simulink model "hilTest"  (R2019b)
settings: Solver=ode1  StartTime=0.0  StopTime=Inf  FixedStep=0.001  RelTol=1e-3
PostLoadFcn:
  | , if any(exist('dsrtsu_mdlpostloadfcn', 'file') ~= 0), dsrtsu_mdlpostloadfcn('Execute', bdroot); end,
InitFcn:
  | , if any(exist('rtifpga_mdlclblib', 'file') ~= 0), rtifpga_mdlclblib('Init', bdroot); end,
undefined symbols (not defined in the file or in its folder): rticanmm_blockfcn, rticanmm_initfcn
libraries: rtimmsu_dsrtlib x2
Description:
  | Standard RTI1006 template.
  | Supported MATLAB version:  R2019b.
settings Model: Tag=RTI1006  DSRTSU_INTERNAL_RTI_VER=560  DSRTSU_INTERNAL_RTI_TYPE=rti1006  RTICANMMDATA=struct('GeneralSetupData',struct('modelroot','C:\Users\uweco\Desktop\Git\ArudinoCANDisplay\HIL','generalsettings',struct('filesettings',struct('destfolder',struct('Name','RTICANMM_FILES','Check',1),'buildfolder',struct('Name','.','Check',1),'AbsDestfolder',struct('Name','C:\Users\uweco\Desktop\Git\ArudinoCANDisplay\HIL\RTICANMM_FILES'),'AbsBuildfolder',struct('Name','C:\Users\uweco\Desktop\Git\ArudinoCANDisplay\HIL'))),'options',struct('addpaths',1,'rmpaths',1,'addtrcexclusion',1,'cannavigator',struct('checkmonitoring',1),'show_usrtrc',0,'use_usrtrc',0,'addpath2usrmk',1,'disableclosing',0),'advanced',struct('options',ones(1,100)),'MPSetup',{{}},'modelname','hilTest','blockdata',struct('generalsettings',struct('filesettings',struct('destfolder',struct('Name','.','Check',1),'AbsDestfolder',struct('Name','T:\TOOL_SOURCES\CANnedy\m'),'buildfolder',struct('Name','.','Check',1),'AbsBuildfolder',struct('Name','C:\MATLAB6p5\work'))),'options',struct('addpaths',1,'rmpaths',1,'addpath2usrmk',1),'modelname','rticanmmlib','modelroot','T:\TOOL_SOURCES\CANnedy\m'),'MMType','RTICANMM','block',['hilTest/RTICANMM' char(10) 'GeneralSetup'],'RTI',struct('Type','RTI1006','Ver','7.14','Date','02-May-2020'),'version','5.4.737888.359837963','userdata',struct('HostServiceChannelID',{{'CAVPCM'}})))  DSRTSU_INTERNAL_RTIFPGA=160  Creator=uweco  LastModifiedBy=uweco
settings DataIOCC: ReturnWorkspaceOutputs=off
settings OptimizationCC: BlockReduction=off  OptimizeBlockIOStorage=off  BufferReuse=off  GlobalBufferReuse=off  ExpressionFolding=off  LocalBlockOutputs=off  OptimizeDataStoreBuffers=off  BusAssignmentInplaceUpdate=off
settings DebuggingCC: PregeneratedLibrarySubsystemCodeDiagnostic=none  ArithmeticOperatorsInVariantConditions=warning
settings HardwareCC: ProdBitPerPointer=32  ProdBitPerSizeT=32  ProdBitPerPtrDiffT=32  ProdLargestAtomicInteger=Integer  ProdWordSize=32  ProdLongLongMode=on  ProdHWDeviceType=Custom Processor->Custom  TargetIntDivRoundTo=Zero  TargetEndianess=LittleEndian  TargetHWDeviceType=Custom Processor->Custom
settings ModelReferenceCC: EnableParallelModelReferenceBuilds=on  ParallelModelReferenceMATLABWorkerInit=Load Top Model
settings SFSimCC: SimUseLocalCustomCode=off  MATLABDynamicMemAlloc=off  CustomCodeUndefinedFunction=UseInterfaceOnly
settings RTWCC: Description=dSPACE DS1006 Hardware Platform  SystemTargetFile=rti1006.tlc  MakeCommand=make_rti  TemplateMakefile=rti1006.tmf  RTWUseLocalCustomCode=off
settings CodeAppCC: StateflowObjectComments=on
settings STFCustomTargetCC: ParMdlRefBuildCompliant=on  SystemTargetFile=rti1006.tlc
settings GRTTargetCC: TargetLangStandard=C89/C90 (ANSI)  CompOptLevelCompliant=off  ConcurrentExecutionCompliant=off  CombineOutputUpdateFcns=off  MatFileLogging=off  CPPClassGenCompliant=off  UseToolchainInfoCompliant=off
settings ConfigComp: CovMetricSettings=dswe

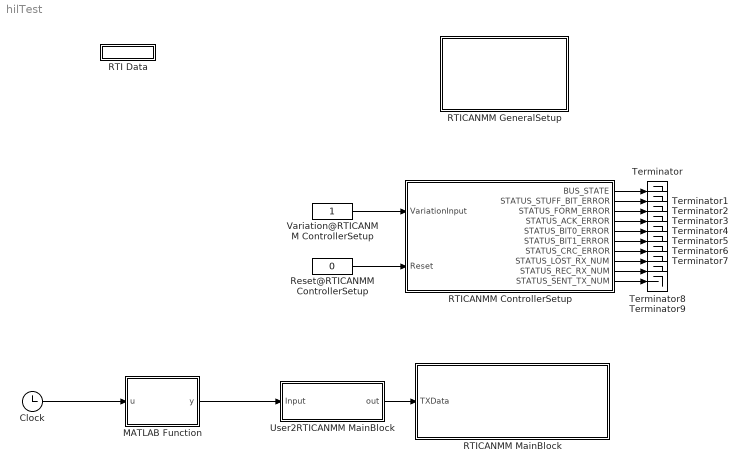
== system hilTest ==
  Clock : Clock
  MATLAB Function : MATLAB Function  TreatAsAtomicUnit=on
  RTI Data : Subsystem  Tag=struct('RTIDataServer',struct('RTIDataServerVs','2','RTIModelDescription','struct(''main'',''hilTest'',''sub'','''',''isMp'',0)'))  LoadFcn="if exist('rtidc'), try,  rtidc('DataHostBlockClbLoad', gcbh); catch, disp(['Warning: ''LoadFcn'' for RTI Data block failed: ' lasterr]); end, end,"  mask(RTI_DATA_HOST){}
      mask help:
      | RTI Data Block.
      | This block is used by RTI to store internal model-dependent data.
      | Please keep this block on the root level of the model. Deleting this block will result in data loss.
      |
      | NEVER DELETE OR COPY THIS BLOCK!
      settings: CopyFcn="if exist('rtidc'), try,  rtidc('DataHostBlockClbCopy', gcbh); catch, disp(['Warning: ''CopyFcn'' for RTI Data block failed: ' lasterr]); end, end,"  DeleteFcn="if exist('rtidc'), try,  rtidc('DataHostBlockClbDelete', gcbh); catch, disp(['Warning: ''DeleteFcn'' for RTI Data block failed: ' lasterr]); end, end,"  ModelCloseFcn="if exist('rtidc'), try,  rtidc('DataHostBlockClbModelClose', gcbh); catch, disp(['Warning: ''ModelCloseFcn'' for RTI Data block failed: ' lasterr]); end, end,"  PreSaveFcn="if exist('rtidc'), try,  rtidc('DataHostBlockClbPreSave', gcbh); catch, disp(['Warning: ''PreSaveFcn'' for RTI Data block failed: ' lasterr]); end, end,"  PostSaveFcn="if exist('rtidc'), try,  rtidc('DataHostBlockClbPostSave', gcbh); catch, disp(['Warning: ''PostSaveFcn'' for RTI Data block failed: ' lasterr]); end, end,"  NameChangeFcn="if exist('rtidc'), try,  rtidc('DataHostBlockClbNameChange', gcbh); catch, disp(['Warning: ''NameChangeFcn'' for RTI Data block failed: ' lasterr]); end, end,"
      mask Help:
      | RTI Data Block.
      | This block is used by RTI to store internal model-dependent data.
      | Please keep this block on the root level of the model. Deleting this block will result in data loss.
      | 
      | NEVER DELETE OR COPY THIS BLOCK!
      mask Display:
      | text(0.5, 0.5, 'RTI Data', 'HorizontalAlignment', 'center');
      | plot([1 0]);
  RTICANMM ControllerSetup : Subsystem  InitFcn=rticanmm_blockfcn('InitFcn', 'CANnedySetup', gcb)  ClipboardFcn=rticanmm_blockfcn('ClipboardFcn', 'CANnedySetup', gcb)  mask(RTICANMM){DSProperties=struct('RTI',struct('Version',uint32(1),'BlockType',struct('isSLSource',uint8(1),'isSLSink',uint8(1),'isHWSource',uint8(0),'isHWSink',uint8(0),'isSetup',uint8(0),'isInline',uint8(1),'isNonInline',uint8(0),'isInterrupt',uint8(0),'isChannelwise',uint8(0)),'IOBoardType','RTICANMM','UnitType','RTICANMM','Identifier','BUSSETUP','DialogType','SL','BlockSet','RTICANMM','SlaveProcessor','CAN')), CANMMProperties=struct('cannedy',struct('data',struct('options',struct('controllername','CAVPCM','controllernameautomatic',[],'loglevel','0','checkrealtime',0,'checkchangebaudrate',0,'sampletime','1.000','CANControllerStatus',1,'NumberofStuffErr',1,'NumberofFormErr',1,'NumberofAckErr',1,'NumberofBit0Err',1,'NumberofsuccrecRX',1,'Numberofsuccsent',1,'NumberofBit1Err',1,'NumberofCRCErr',1,'NumberoflostRX',1,'Busoff',0,'Busload',0,'OperationPending',0,'TxRetryCount',3,'addtrcexclusion',true,'cannavigator',struct('checkmonitoring',0,'checkinternmonitoring',0),'show_usrtrc',0,'use_usrtrc',0,'checkchangebaudrateFD',0,'errorframegeneration',0,'efgenabled',0),'modelroot','C:\Users\uweco\Desktop\Git\ArudinoCANDisplay\HIL','generalsettings',struct('setupdata',struct('board','DS2202','boardno',1,'channelno',1,'Type','STD','transceiver','ISO11898-2','busconfig','0x0','feedthrough','false','resistance',struct('r120',1,'roff',0,'r16',1,'r10',0),'baudrate','500','Frequency',[24 36],'samplemode',1,'commChannelTJA1041',6,'config',struct('standard',1,'advanced',0,'register',struct('btr0','0x41','btr1','0x1E','sp','88','sjw','1','tseg1','14','tseg2','1','brp','1','smpl','0','btr0_36','0x41','btr1_36','0x1E','sp_36','88','sjw_36','1','tseg1_36','14','tseg2_36','1','brp_36','1','smpl_36','0','btr0_64','0x41','btr1_64','0x1E','sp_64','88','sjw_64','1','tseg1_64','14','tseg2_64','1','brp_64','1','smpl_64','0')),'channelcfg',struct('INTENDISABLE','CAN_INT_DISABLE','intenable',0),'SETUPID','RTICANMM_CAVPCM_ID','CONTROLLER_ID','CANMM_CTL_SETUP_CAVPCM','mainblock_includefile','RTICANMM_SETUP_CAVPCM','canfdenable',0,'canfdboardselected',0,'slotno',1,'moduletype','DS4342','baudrateFD','4000','samplePoint','80','samplePointFD','80','termination','TERMINATION_ON'),'filesettings',struct('destfolder',struct('Name','RTICANMM_FILES','Check',1),'buildfolder',struct('Name','.','Check',1))),'advanced',struct('options',ones(1,100)),'partialnetdata',struct('switchedon',0,'format','STD','idmask',['XXXXX XXXXXXXX XXXXXXXX XXXXXXXX'],'idcode','0','idfilter','0','datamaskused',0,'datalength','0','datamask','0x0000000000000000','partialnetworkenable',0)),'blk',['hilTest/RTICANMM' char(10) 'ControllerSetup'],'allgeneratedfiles',{{'C:\Users\uweco\Desktop\Git\ArudinoCANDisplay\HIL\RTICANMM_FILES\RTICANMM_SETUP_CAVPCM.c','C:\Users\uweco\Desktop\Git\ArudinoCANDisplay\HIL\RTICANMM_FILES\RTICANMM_SETUP_CAVPCM.h','c:\users\uweco\desktop\git\arudinocandisplay\hil\rticanmm_files\rticanmm_setup_cavpcm.mexw64'}},'ismp',false,'BlockDataVersion','0.9.0','recreate',0),'CANnedynew',0,'CANnedySettings','CAVPCM','GeneratedFiles',{{'C:\Users\uweco\Desktop\Git\ArudinoCANDisplay\HIL\RTICANMM_FILES\RTICANMM_SETUP_CAVPCM.c','C:\Users\uweco\Desktop\Git\ArudinoCANDisplay\HIL\RTICANMM_FILES\RTICANMM_SETUP_CAVPCM.h','c:\users\uweco\desktop\git\arudinocandisplay\hil\rticanmm_files\rticanmm_setup_cavpcm.mexw64'}},'SFCN','RTICANMM_SETUP_CAVPCM.c','HostService',struct('Tags',struct('DATA','RTICANMM_MonitorData','TimeStampGlobal','RTICANMM_MonitoringTimeStamp','TimeStampGlobalEnable','RTICANMM_MonitoringTimeStampEnable','Enable','CANMMMonitor_CAVPCM','TimeStamp','MonitoringTimeStamp_CAVPCM'),'DATA',struct('Length',18),'Info',struct('Desc',{'ID','Service','Data1','Data2','Data3','Data4','Data5','Data6','Data7','Data8','Data9','Data10','Data11','Data12','Data13','Data14','Data15','Data16'}),'Names',struct('TimeStampGlobal','TimeStamp','TimeStampGlobalEnable','TimeStamp_Enable','Enable','Monitoring_Enable','TimeStamp','Monitoring_TimeStamp'),'ChannelID',1)), CANMMType=CANnedySetup, CANMMFolder=C:\Users\uweco\Desktop\Git\ArudinoCANDisplay\HIL, CANMMDestFolder=RTICANMM_FILES, CANMMSettings=CAVPCM, CANMMSFcn=RTICANMM_SETUP_CAVPCM, CANMMBoard=DS2202, CANMMBoardNum=1, CANMMChannel=1}
      settings: AttributesFormatString=%<CANMMSettings>: %<CANMMBoard>_B%<CANMMBoardNum>_C%<CANMMChannel>  CopyFcn=rticanmm_blockfcn('CopyFcn', 'CANnedySetup', gcb)  DeleteFcn=rticanmm_blockfcn('DeleteFcn', 'CANnedySetup', gcb)  ModelCloseFcn=rticanmm_blockfcn('ModelCloseFcn', 'CANnedySetup', gcb)  NameChangeFcn=rticanmm_blockfcn('NameChangeFcn', 'CANnedySetup', gcb)  OpenFcn=try, rticanmm_setup_gui('create',gcb); ; catch,errordlg({lasterr, '','Please check your RTI installation.'},['Error: ' upper(bdroot)], 'replace'); end  MoveFcn=rticanmm_blockfcn('MoveFcn', 'CANnedySetup', gcb)
      mask Help: eval('rticanmm_quickstart(''create'', gcb);', 'disp(lasterr);')
      mask Display:
      | disp('RTI CAN\nMultiMessage\nControllerSetup')
      | 
      | port_label('input', 1 , 'Variation')
      | port_label('input', 2 , 'Reset')
      | port_label('output', 1, 'Status')
      | port_label('output', 2, 'Stuff errors')
      | port_label('output', 3, 'Format errors')
      | port_label('output', 4, 'Ack errors')
      | port_label('output', 5, 'Bit 0 errors')
      | port_label('output', 6, 'Bit 1 errors')
      | port_label('output', 7, 'CRC errors')
      | port_label('output', 8, 'RX lost')
      | port_label('output', 9, 'RX ok')
      | port_label('output', 10, 'TX ok')
  RTICANMM GeneralSetup : Subsystem  InitFcn=rticanmm_initfcn(gcb, 'CANnedySettings')  ClipboardFcn=rticanmm_blockfcn('ClipboardFcn', 'CANnedySettings', gcb)  mask(RTICANMM){DSProperties=struct('RTI',struct('Version',uint32(1),'BlockType',struct('isSLSource',uint8(1),'isSLSink',uint8(1),'isHWSource',uint8(0),'isHWSink',uint8(0),'isSetup',uint8(0),'isInline',uint8(1),'isNonInline',uint8(0),'isInterrupt',uint8(0),'isChannelwise',uint8(0)),'IOBoardType','RTICANMM','UnitType','RTICANMM','Identifier','GENERALSETUP','DialogType','SL','BlockSet','RTICANMM','SlaveProcessor','CAN')), CANMMDestFolder=RTICANMM_FILES, CANMMBuildDir=., CANMMAddPaths=on, CANMMAddpathUserMake=on, CANMMRemovePathOnclose=on, CANMMType=CANnedySettings, CANMMProperties=struct('modelroot','C:\Users\uweco\Desktop\Git\ArudinoCANDisplay\HIL','generalsettings',struct('filesettings',struct('destfolder',struct('Name','RTICANMM_FILES','Check',1),'buildfolder',struct('Name','.','Check',1),'AbsDestfolder',struct('Name','C:\Users\uweco\Desktop\Git\ArudinoCANDisplay\HIL\RTICANMM_FILES'),'AbsBuildfolder',struct('Name','C:\Users\uweco\Desktop\Git\ArudinoCANDisplay\HIL'))),'options',struct('addpaths',1,'rmpaths',1,'addtrcexclusion',1,'cannavigator',struct('checkmonitoring',1),'show_usrtrc',0,'use_usrtrc',0,'addpath2usrmk',1,'disableclosing',0),'advanced',struct('options',ones(1,100)),'MPSetup',{{}},'modelname','hilTest','blockdata',struct('generalsettings',struct('filesettings',struct('destfolder',struct('Name','.','Check',1),'AbsDestfolder',struct('Name','T:\TOOL_SOURCES\CANnedy\m'),'buildfolder',struct('Name','.','Check',1),'AbsBuildfolder',struct('Name','C:\MATLAB6p5\work'))),'options',struct('addpaths',1,'rmpaths',1,'addpath2usrmk',1),'modelname','rticanmmlib','modelroot','T:\TOOL_SOURCES\CANnedy\m'),'MMType','RTICANMM','block',['hilTest/RTICANMM' char(10) 'GeneralSetup'],'RTI',struct('Type','RTI1006','Ver','7.14','Date','02-May-2020'),'version','5.4.737888.359837963','userdata',struct('HostServiceChannelID',{{'CAVPCM'}}))}
      mask prompts: CANMMDestFolder "Destination Folder for generated Files:"; CANMMBuildDir "Build Directory (*_usr.mk, *_usr.trc)"; CANMMAddPaths "Add Paths automatically"; CANMMAddpathUserMake "Add Paths to UserMake-File"; CANMMRemovePathOnclose "Remove added Path on ModelClose"
      mask init:
      | rticanmm_initfcn(gcb,'CANnedyGeneralSettings')
      settings: CopyFcn=rticanmm_blockfcn('CopyFcn', 'CANnedySettings', gcb)  DeleteFcn=rticanmm_blockfcn('DeleteFcn', 'CANnedySettings', gcb)  ModelCloseFcn=rticanmm_blockfcn('CloseFcn', 'CANnedyGeneralSettings', gcb)  NameChangeFcn=rticanmm_blockfcn('NameChangeFcn', 'CANnedySettings', gcb)  OpenFcn=try, rticanmm_gs_gui('create',gcb), ; catch,errordlg({lasterr, '','Please check your RTI installation.'},['Error: ' upper(bdroot)], 'replace'); end  MoveFcn=rticanmm_blockfcn('MoveFcn', 'CANnedySettings', gcb)
      mask Help: eval('rticanmm_quickstart(''create'', gcb);', 'disp(lasterr);')
      mask Display: disp(sprintf(['RTI CAN\nMultiMessage\nGeneralSetup']))
  RTICANMM MainBlock : Subsystem  InitFcn=rticanmm_blockfcn('InitFcn', 'CANnedy', gcb)  ClipboardFcn=rticanmm_blockfcn('ClipboardFcn', 'CANnedy', gcb)  mask(RTICANMM){DSProperties=struct('RTI',struct('Version',uint32(1),'BlockType',struct('isSLSource',uint8(1),'isSLSink',uint8(1),'isHWSource',uint8(0),'isHWSink',uint8(0),'isSetup',uint8(0),'isInline',uint8(1),'isNonInline',uint8(0),'isInterrupt',uint8(0),'isChannelwise',uint8(0)),'IOBoardType','RTICANMM','UnitType','RTICANMM','Identifier','Mainblock','DialogType','SL','BlockSet','RTICANMM','SlaveProcessor','CAN')), CANMMProperties=struct('RTICANMMVersion','5.4','RTICANMMVersionIntern','5.4.737888.359837963','RTICANMMDate','02-May-2020','Settings','RTICANMM_MAIN_CAN','UserTracePath','','ModelPath','C:\Users\uweco\Desktop\Git\ArudinoCANDisplay\HIL','filesettings',struct('FileName','EMC_PCM_CAV_Interface.dbc','IsRelative',1,'ClusterId',1,'ClusterList',{{'default'}},'destfolder',struct('Name','RTICANMM_FILES','Check',1),'buildfolder',struct('Name','.','Check',1),'onlyfreerawcapture',0,'overlapping2variant',0,'canfdsupport',0,'shortestJ2container',1),'onlyfreerawcapture',0,'Board','DS2202','BoardNum','1','ChannelNum','1','Variation','1','SetupId','CAVPCM','MARK',['2F41AF6EC10DA9912F13F480927801';'3F2E6D3DFA4E4E3DB249B5E653EB56';'4BC74496B8D903D68E6C1CC355777E';'0871956A691268807472F04F47193C';'5047585669399549A211899E4AA71C'],'date','02-May-2022','clock',['02.05.2022 10:07:20'],'recreate',0,'RTIVER','RTI1006','j1939',0,'TRC',struct('include',1),'rtsupport',struct('XMLFile','C:\Users\uweco\Desktop\Git\ArudinoCANDisplay\HIL\RTICANMM_FILES\RTICANMM_MAIN_CAN.xml','DBCXML',struct('Path','C:\Users\uweco\Desktop\Git\ArudinoCANDisplay\HIL\RTICANMM_FILES\RTICANMM_MAIN_CAN_dbc.xml','support',1,'Name','EMC_PCM_CAV_Interface.dbc','Date',['27-Apr-2022 10:21:25'],'Type','standard','DBCSupport','ON'))), CANMMType=CANnedy, CANMMUserTraceMerged=off, CANMMUserTracePath=, CANMMChannelNum=1, CANMMBoardNum=1, CANMMDestFolder=RTICANMM_FILES, CANMMFolder=., CANMMSetupId=CAVPCM, CANMMsave2mat=['2F41AF6EC10DA9912F13F480927801';'3F2E6D3DFA4E4E3DB249B5E653EB56';'4BC74496B8D903D68E6C1CC355777E';'0871956A691268807472F04F47193C';'5047585669399549A211899E4AA71C'], CANMMName=CAN, CANMMSettings=RTICANMM_MAIN_CAN, CANMMIntermediateTag=RTICANMM_MAIN_CAN_intermediate, CANMMsfcnname=RTICANMM_MAIN_CAN}
      mask init:
      | rticanmm_initfcn(gcb, CANMMType, CANMMsfcnname)
      settings: AttributesFormatString=CAVPCM[CAN]: DS2202_B1_C1_V1  CopyFcn=rticanmm_blockfcn('CopyFcn', 'CANnedy', gcb)  DeleteFcn=rticanmm_blockfcn('DeleteFcn', 'CANnedy', gcb)  ModelCloseFcn=rticanmm_blockfcn('ModelCloseFcn', 'CANnedy', gcb)  NameChangeFcn=rticanmm_blockfcn('NameChangeFcn', 'CANnedy', gcb)  OpenFcn=try, rticanmm_main_gui('create',gcb); ; catch,errordlg({lasterr, '','Please check your RTI installation.'},['Error: ' upper(bdroot)], 'replace'); end  MoveFcn=rticanmm_blockfcn('MoveFcn', 'CANnedy', gcb)
      mask Help: eval('rticanmm_quickstart(''create'', gcb);', 'disp(lasterr);')
      mask Display:
      | disp(sprintf('RTI CAN\nMultiMessage\nMainBlock'))
      | port_label('input', 1, 'TX Data')
  Reset@RTICANMM ControllerSetup : Constant  Value=0  OutDataTypeStr=boolean
  Terminator{,1..9} (10 alike) : Terminator
  User2RTICANMM MainBlock : Subsystem
      mask Display: disp('Mapping\nto RTICANMM')
  Variation@RTICANMM ControllerSetup : Constant  OutDataTypeStr=uint8
  wires:
  Variation@RTICANMM ControllerSetup/1 -> RTICANMM ControllerSetup/1(VariationInput)
  Reset@RTICANMM ControllerSetup/1 -> RTICANMM ControllerSetup/2(Reset)
  User2RTICANMM MainBlock/1(out) -> RTICANMM MainBlock/1(TXData)
  Clock/1 -> MATLAB Function/1(u)
  MATLAB Function/1(y) -> User2RTICANMM MainBlock/1(Input)
  RTICANMM ControllerSetup/1(BUS_STATE) -> Terminator/1
  RTICANMM ControllerSetup/2(STATUS_STUFF_BIT_ERROR) -> Terminator1/1
  RTICANMM ControllerSetup/3(STATUS_FORM_ERROR) -> Terminator2/1
  RTICANMM ControllerSetup/4(STATUS_ACK_ERROR) -> Terminator3/1
  RTICANMM ControllerSetup/5(STATUS_BIT0_ERROR) -> Terminator4/1
  RTICANMM ControllerSetup/6(STATUS_BIT1_ERROR) -> Terminator5/1
  RTICANMM ControllerSetup/7(STATUS_CRC_ERROR) -> Terminator6/1
  RTICANMM ControllerSetup/8(STATUS_LOST_RX_NUM) -> Terminator7/1
  RTICANMM ControllerSetup/9(STATUS_REC_RX_NUM) -> Terminator8/1
  RTICANMM ControllerSetup/10(STATUS_SENT_TX_NUM) -> Terminator9/1

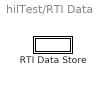
== system hilTest/RTI Data ==
  RTI Data Store : Subsystem  Tag="struct('public',struct('sub',struct('name',{{'hilTest'}},'data',{{struct('TH',struct('thTaskInfo',struct('taskType',{'TIMER','HWINT','TMRINT','SWINT','GLINT'},'tasksNumOf',{1,0,0,0,0},'srcIds',{{'TIMERA'},{},{},{},{}},'taskNames',{{['Timer Task 1']},{},{},{},{}})),'th_tc',struct('dataType','TASK','taskGroupId','','taskGroupList',{{}},'taskSchedulingPolicy','FCFS','taskType','TIMER','blkh',-1,'srcId','TIMERA','srcSgnName',['Timer A interrupt'],'srcCpuName','','taskName',['Timer Task 1  [0.001] s'],'taskNameDisplayExt','','smplTime',0.001,'smplTimeOffs',0,'hasFixedPriority',0,'priority',1,'hasFixedOvc',0,'ovcType',1,'ovcMax',1),'tc_th',struct('dataType','TASK','taskGroupId','','taskGroupList',{{}},'taskSchedulingPolicy','FCFS','taskType','TIMER','blkh',-1,'srcId','TIMERA','srcSgnName',['Timer A interrupt'],'srcCpuName','','taskName',['Timer Task 1  [0.001] s'],'taskNameDisplayExt','','smplTime',0.001,'smplTimeOffs',0,'hasFixedPriority',0,'priority',1,'hasFixedOvc',0,'ovcType',1,'ovcMax',1))}})),'private',struct('version',struct('dsVer',uint32(2)),'access',struct('modified',['02-May-2022 10:17:38'],'type','Model','isPerm',1)))"  mask(RTI_DATA_STORE){}
      mask help:
      | RTI Data Store Block. This block is used by RTI to store internal model dependent data. Deleting this block will result in data loss.
      |
      | NEVER DELETE, COPY, OR MODIFY THIS BLOCK!
      mask Help:
      | RTI Data Store Block. This block is used by RTI to store internal model dependent data. Deleting this block will result in data loss.
      | 
      | NEVER DELETE, COPY, OR MODIFY THIS BLOCK!
      mask Display: text(0.5, 0.5, ' ', 'HorizontalAlignment', 'center');

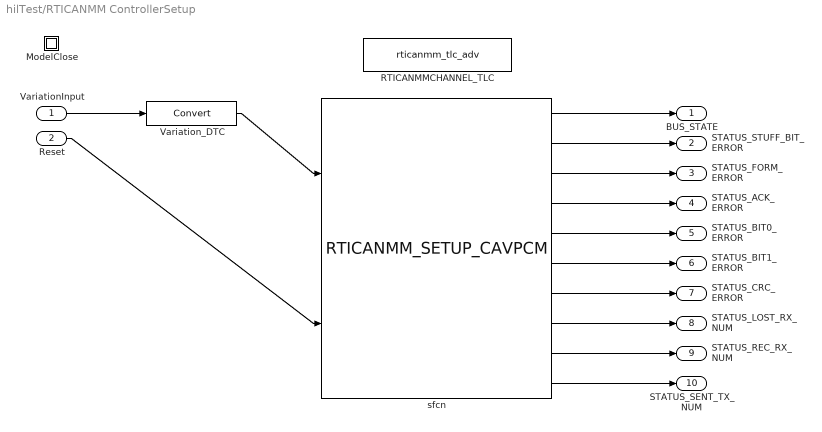
== system hilTest/RTICANMM ControllerSetup ==
  VariationInput : Inport
  Reset : Inport  Port=2
  ModelClose : Subsystem  mask(RTICANMMModelClose){}
  RTICANMMCHANNEL_TLC : S-Function  FunctionName=rticanmm_tlc_adv  Parameters=2202,1,1,0,500,22021143421  SFunctionDeploymentMode=off  EnableBusSupport=off  mask(RTICANMMCHANNEL_TLC){}
  Variation_DTC : DataTypeConversion  SaturateOnIntegerOverflow=on  RndMeth=Zero
  sfcn : S-Function  InitFcn=rticanmm_initfcn(gcb, 'SFCNs')  FunctionName=RTICANMM_SETUP_CAVPCM  SFunctionDeploymentMode=off  EnableBusSupport=off
      mask init:
      | rticanmm_initfcn(gcb, 'SFCNs')
  BUS_STATE : Outport
  STATUS_STUFF_BIT_ERROR : Outport  Port=2
  STATUS_FORM_ERROR : Outport  Port=3
  STATUS_ACK_ERROR : Outport  Port=4
  STATUS_BIT0_ERROR : Outport  Port=5
  STATUS_BIT1_ERROR : Outport  Port=6
  STATUS_CRC_ERROR : Outport  Port=7
  STATUS_LOST_RX_NUM : Outport  Port=8
  STATUS_REC_RX_NUM : Outport  Port=9
  STATUS_SENT_TX_NUM : Outport  Port=10
  wires:
  Reset/1 -> sfcn/2
  sfcn/1 -> BUS_STATE/1
  sfcn/2 -> STATUS_STUFF_BIT_ERROR/1
  sfcn/3 -> STATUS_FORM_ERROR/1
  sfcn/4 -> STATUS_ACK_ERROR/1
  sfcn/5 -> STATUS_BIT0_ERROR/1
  sfcn/6 -> STATUS_BIT1_ERROR/1
  sfcn/7 -> STATUS_CRC_ERROR/1
  sfcn/8 -> STATUS_LOST_RX_NUM/1
  sfcn/9 -> STATUS_REC_RX_NUM/1
  sfcn/10 -> STATUS_SENT_TX_NUM/1
  VariationInput/1 -> Variation_DTC/1
  Variation_DTC/1 -> sfcn/1

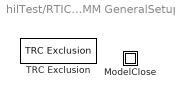
== system hilTest/RTICANMM GeneralSetup ==
  ModelClose : Subsystem  mask(RTICANMMModelClose){}
  TRC Exclusion : rtimmsu_dsrtlib/TRC Exclusion

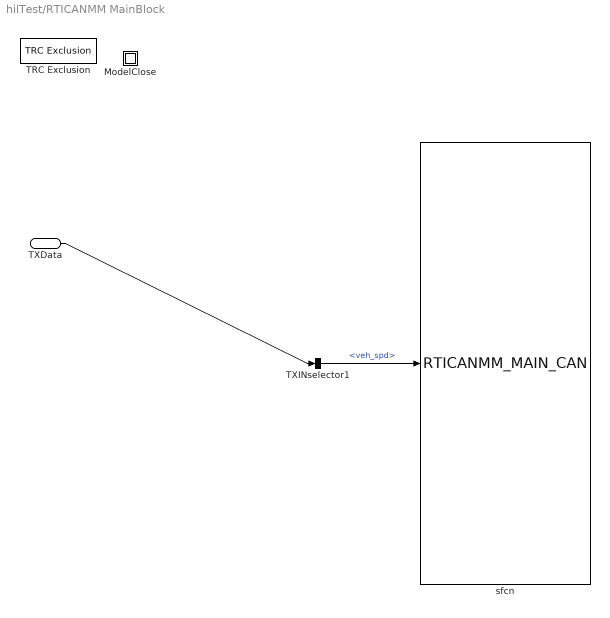
== system hilTest/RTICANMM MainBlock ==
  TXData : Inport
  ModelClose : Subsystem  mask(RTICANMMModelClose){}
  TRC Exclusion : rtimmsu_dsrtlib/TRC Exclusion
  TXINselector1 : BusSelector  OutputSignals=PcmToCav1.veh_spd
  sfcn : S-Function  InitFcn=rticanmm_initfcn(gcb, 'SFCNs')  FunctionName=RTICANMM_MAIN_CAN  SFunctionDeploymentMode=off  EnableBusSupport=off
      mask init:
      | rticanmm_initfcn(gcb, 'SFCNs')
  wires:
  TXData/1 -> TXINselector1/1
  TXINselector1/1 -> sfcn/1  "<veh_spd>"

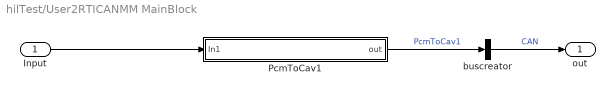
== system hilTest/User2RTICANMM MainBlock ==
  Input : Inport
  PcmToCav1 : Subsystem
  buscreator : BusCreator  Inputs=1
  out : Outport
  wires:
  PcmToCav1/1(out) -> buscreator/1  "PcmToCav1"
  buscreator/1 -> out/1  "CAN"
  Input/1 -> PcmToCav1/1(In1)

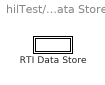
== system hilTest/RTI Data/RTI Data Store ==
  RTI Data Store : Subsystem  mask(RTI_DATA_STORE){}
      mask help:
      | RTI Data Store Block. This block is used by RTI to store internal model dependent data. Deleting this block will result in data loss.
      |
      | NEVER DELETE, COPY, OR MODIFY THIS BLOCK!
      mask Help:
      | RTI Data Store Block. This block is used by RTI to store internal model dependent data. Deleting this block will result in data loss.
      | 
      | NEVER DELETE, COPY, OR MODIFY THIS BLOCK!
      mask Display: text(0.5, 0.5, ' ', 'HorizontalAlignment', 'center');

== system hilTest/RTICANMM ControllerSetup/ModelClose ==

== system hilTest/RTICANMM GeneralSetup/ModelClose ==

== system hilTest/RTICANMM MainBlock/ModelClose ==

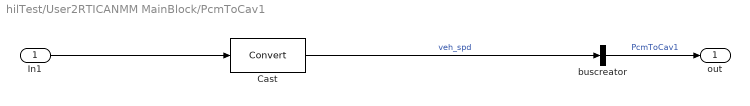
== system hilTest/User2RTICANMM MainBlock/PcmToCav1 ==
  In1 : Inport
  Cast : DataTypeConversion
  buscreator : BusCreator  Inputs=1
  out : Outport
  wires:
  buscreator/1 -> out/1  "PcmToCav1"
  Cast/1 -> buscreator/1  "veh_spd"
  In1/1 -> Cast/1

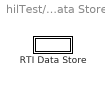
== system hilTest/RTI Data/RTI Data Store/RTI Data Store ==
  RTI Data Store : Subsystem  mask(RTI_DATA_STORE){}
      mask help:
      | RTI Data Store Block. This block is used by RTI to store internal model dependent data. Deleting this block will result in data loss.
      |
      | NEVER DELETE, COPY, OR MODIFY THIS BLOCK!
      mask Help:
      | RTI Data Store Block. This block is used by RTI to store internal model dependent data. Deleting this block will result in data loss.
      | 
      | NEVER DELETE, COPY, OR MODIFY THIS BLOCK!
      mask Display: text(0.5, 0.5, ' ', 'HorizontalAlignment', 'center');

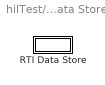
== system hilTest/RTI Data/RTI Data Store/RTI Data Store/RTI Data Store ==
  RTI Data Store : Subsystem  mask(RTI_DATA_STORE){}
      mask help:
      | RTI Data Store Block. This block is used by RTI to store internal model dependent data. Deleting this block will result in data loss.
      |
      | NEVER DELETE, COPY, OR MODIFY THIS BLOCK!
      mask Help:
      | RTI Data Store Block. This block is used by RTI to store internal model dependent data. Deleting this block will result in data loss.
      | 
      | NEVER DELETE, COPY, OR MODIFY THIS BLOCK!
      mask Display: text(0.5, 0.5, ' ', 'HorizontalAlignment', 'center');

== system hilTest/RTI Data/RTI Data Store/RTI Data Store/RTI Data Store/RTI Data Store ==

== matlab function hilTest/MATLAB Function ==
  data: u input; y output
function y = fcn(u)

y = mod(u, 69);
